simulink model "controller2"  (R2018a)
settings: Solver=VariableStepAuto  StartTime=0.0  StopTime=10.0  RelTol=1e-3
undefined symbols (not defined in the file or in its folder): quant
settings Model: Creator=lixinru  LastModifiedBy=lixinru

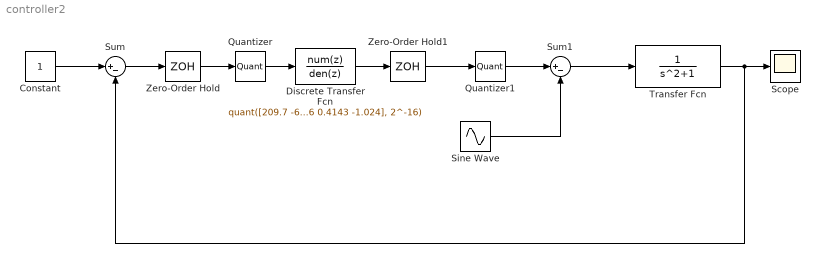
== system controller2 ==
  Constant : Constant
  Discrete Transfer Fcn : DiscreteTransferFcn  Numerator=quant([209.7 -671.5 954.7 -693.3 204.8], 2^-16)  Denominator=quant([1 -0.3099 -0.5444 0.4636 0.4143 -1.024], 2^-16)
  Quantizer : Quantizer  QuantizationInterval=0.01
  Quantizer1 : Quantizer  QuantizationInterval=0.01
  Scope : Scope
  Sine Wave : Sin  Frequency=10  SampleTime=0
  Sum : Sum  Inputs=|+-
  Sum1 : Sum  Inputs=|+-
  Transfer Fcn : TransferFcn  Denominator=[1 0 1]
  Zero-Order Hold : ZeroOrderHold  SampleTime=0.1
  Zero-Order Hold1 : ZeroOrderHold  SampleTime=-1
  wires:
  Zero-Order Hold1/1 -> Quantizer1/1
  Transfer Fcn/1 -> Sum/2, Scope/1
  Discrete Transfer Fcn/1 -> Zero-Order Hold1/1
  Quantizer/1 -> Discrete Transfer Fcn/1
  Quantizer1/1 -> Sum1/1
  Zero-Order Hold/1 -> Quantizer/1
  Constant/1 -> Sum/1
  Sum1/1 -> Transfer Fcn/1
  Sum/1 -> Zero-Order Hold/1
  Sine Wave/1 -> Sum1/2
